simulink model "ASDdc_SelectParameter"  (R2016b)
settings: configuration reference "CodeGenConfigSet" (kept outside this file)
values from neighbouring files (symbols this model uses):
  ASDdc_DT1GovGear0_CUR = Calibration.Parameter    [init_ASDdc_SelectParameter.m]    (also in init_ASDdc_SelectParameter_SIL.m = Simulink.Parameter)
  ASDdc_DT1GovGear0_CURX = Calibration.Parameter    [init_ASDdc_SelectParameter.m]    (also in init_ASDdc_SelectParameter_SIL.m = Simulink.Parameter)
  ASDdc_DT1GovGear1_CUR = Calibration.Parameter    [init_ASDdc_SelectParameter.m]    (also in init_ASDdc_SelectParameter_SIL.m = Simulink.Parameter)
  ASDdc_DT1GovGear1_CURX = Calibration.Parameter    [init_ASDdc_SelectParameter.m]    (also in init_ASDdc_SelectParameter_SIL.m = Simulink.Parameter)
  ASDdc_DT1GovGear2_CUR = Calibration.Parameter    [init_ASDdc_SelectParameter.m]    (also in init_ASDdc_SelectParameter_SIL.m = Simulink.Parameter)
  ASDdc_DT1GovGear2_CURX = Calibration.Parameter    [init_ASDdc_SelectParameter.m]    (also in init_ASDdc_SelectParameter_SIL.m = Simulink.Parameter)
  ASDdc_DT1GovGear3_CUR = Calibration.Parameter    [init_ASDdc_SelectParameter.m]    (also in init_ASDdc_SelectParameter_SIL.m = Simulink.Parameter)
  ASDdc_DT1GovGear3_CURX = Calibration.Parameter    [init_ASDdc_SelectParameter.m]    (also in init_ASDdc_SelectParameter_SIL.m = Simulink.Parameter)
  ASDdc_DT1GovGear4_CUR = Calibration.Parameter    [init_ASDdc_SelectParameter.m]    (also in init_ASDdc_SelectParameter_SIL.m = Simulink.Parameter)
  ASDdc_DT1GovGear4_CURX = Calibration.Parameter    [init_ASDdc_SelectParameter.m]    (also in init_ASDdc_SelectParameter_SIL.m = Simulink.Parameter)
  ASDdc_DT1GovGear5_CUR = Calibration.Parameter    [init_ASDdc_SelectParameter.m]    (also in init_ASDdc_SelectParameter_SIL.m = Simulink.Parameter)
  ASDdc_DT1GovGear5_CURX = Calibration.Parameter    [init_ASDdc_SelectParameter.m]    (also in init_ASDdc_SelectParameter_SIL.m = Simulink.Parameter)
  ASDdc_KdGovGear0_CUR = Calibration.Parameter    [init_ASDdc_SelectParameter.m]    (also in init_ASDdc_SelectParameter_SIL.m = Simulink.Parameter)
  ASDdc_KdGovGear0_CURX = Calibration.Parameter    [init_ASDdc_SelectParameter.m]    (also in init_ASDdc_SelectParameter_SIL.m = Simulink.Parameter)
  ASDdc_KdGovGear1_CUR = Calibration.Parameter    [init_ASDdc_SelectParameter.m]    (also in init_ASDdc_SelectParameter_SIL.m = Simulink.Parameter)
  ASDdc_KdGovGear1_CURX = Calibration.Parameter    [init_ASDdc_SelectParameter.m]    (also in init_ASDdc_SelectParameter_SIL.m = Simulink.Parameter)
  ASDdc_KdGovGear2_CUR = Calibration.Parameter    [init_ASDdc_SelectParameter.m]    (also in init_ASDdc_SelectParameter_SIL.m = Simulink.Parameter)
  ASDdc_KdGovGear2_CURX = Calibration.Parameter    [init_ASDdc_SelectParameter.m]    (also in init_ASDdc_SelectParameter_SIL.m = Simulink.Parameter)
  ASDdc_KdGovGear3_CUR = Calibration.Parameter    [init_ASDdc_SelectParameter.m]    (also in init_ASDdc_SelectParameter_SIL.m = Simulink.Parameter)
  ASDdc_KdGovGear3_CURX = Calibration.Parameter    [init_ASDdc_SelectParameter.m]    (also in init_ASDdc_SelectParameter_SIL.m = Simulink.Parameter)
  ASDdc_KdGovGear4_CUR = Calibration.Parameter    [init_ASDdc_SelectParameter.m]    (also in init_ASDdc_SelectParameter_SIL.m = Simulink.Parameter)
  ASDdc_KdGovGear4_CURX = Calibration.Parameter    [init_ASDdc_SelectParameter.m]    (also in init_ASDdc_SelectParameter_SIL.m = Simulink.Parameter)
  ASDdc_KdGovGear5_CUR = Calibration.Parameter    [init_ASDdc_SelectParameter.m]    (also in init_ASDdc_SelectParameter_SIL.m = Simulink.Parameter)
  ASDdc_KdGovGear5_CURX = Calibration.Parameter    [init_ASDdc_SelectParameter.m]    (also in init_ASDdc_SelectParameter_SIL.m = Simulink.Parameter)
settings Model: Creator=lenovo  LastModifiedBy=wangrui
settings ConfigSetRef: SourceLocation=Base Workspace

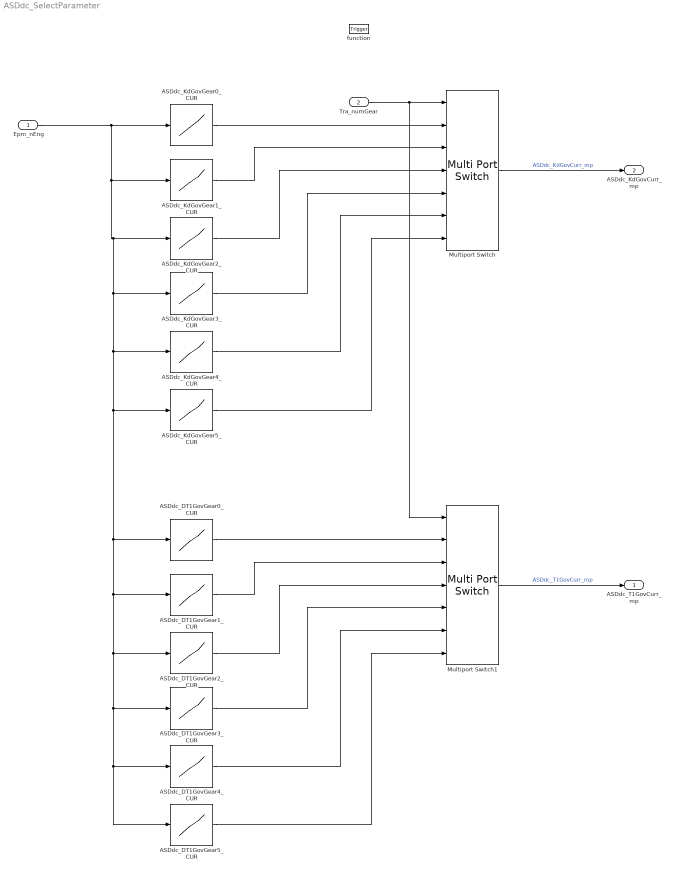
== system ASDdc_SelectParameter ==
  Epm_nEng : Inport  Tag=rpm  Description=Engine speed  OutMin=0  OutMax=6000  OutDataTypeStr=EngSpeed_rpm
  Tra_numGear : Inport  Description=Current gear information  Port=2  OutMin=-128  OutMax=127  OutDataTypeStr=Tra_num
  function : TriggerPort  TriggerType=function-call  VariantControl=Variant
  ASDdc_DT1GovGear0_CUR : Lookup_n-D  NumberOfTableDimensions=1  BreakpointsForDimension1=ASDdc_DT1GovGear0_CURX  IndexSearchMethod=Linear search  BeginIndexSearchUsingPreviousIndexResult=on  Table=ASDdc_DT1GovGear0_CUR  ExtrapMethod=Clip  UseLastTableValue=on  InternalRulePriority=Speed  OutDataTypeStr=Inherit: Inherit via back propagation  SaturateOnIntegerOverflow=on
  ASDdc_DT1GovGear1_CUR : Lookup_n-D  NumberOfTableDimensions=1  BreakpointsForDimension1=ASDdc_DT1GovGear1_CURX  IndexSearchMethod=Linear search  BeginIndexSearchUsingPreviousIndexResult=on  Table=ASDdc_DT1GovGear1_CUR  ExtrapMethod=Clip  UseLastTableValue=on  InternalRulePriority=Speed  OutDataTypeStr=Inherit: Inherit via back propagation  SaturateOnIntegerOverflow=on
  ASDdc_DT1GovGear2_CUR : Lookup_n-D  NumberOfTableDimensions=1  BreakpointsForDimension1=ASDdc_DT1GovGear2_CURX  IndexSearchMethod=Linear search  BeginIndexSearchUsingPreviousIndexResult=on  Table=ASDdc_DT1GovGear2_CUR  ExtrapMethod=Clip  UseLastTableValue=on  InternalRulePriority=Speed  OutDataTypeStr=Inherit: Inherit via back propagation  SaturateOnIntegerOverflow=on
  ASDdc_DT1GovGear3_CUR : Lookup_n-D  NumberOfTableDimensions=1  BreakpointsForDimension1=ASDdc_DT1GovGear3_CURX  IndexSearchMethod=Linear search  BeginIndexSearchUsingPreviousIndexResult=on  Table=ASDdc_DT1GovGear3_CUR  ExtrapMethod=Clip  UseLastTableValue=on  InternalRulePriority=Speed  OutDataTypeStr=Inherit: Inherit via back propagation  SaturateOnIntegerOverflow=on
  ASDdc_DT1GovGear4_CUR : Lookup_n-D  NumberOfTableDimensions=1  BreakpointsForDimension1=ASDdc_DT1GovGear4_CURX  IndexSearchMethod=Linear search  BeginIndexSearchUsingPreviousIndexResult=on  Table=ASDdc_DT1GovGear4_CUR  ExtrapMethod=Clip  UseLastTableValue=on  InternalRulePriority=Speed  OutDataTypeStr=Inherit: Inherit via back propagation  SaturateOnIntegerOverflow=on
  ASDdc_DT1GovGear5_CUR : Lookup_n-D  NumberOfTableDimensions=1  BreakpointsForDimension1=ASDdc_DT1GovGear5_CURX  IndexSearchMethod=Linear search  BeginIndexSearchUsingPreviousIndexResult=on  Table=ASDdc_DT1GovGear5_CUR  ExtrapMethod=Clip  UseLastTableValue=on  InternalRulePriority=Speed  OutDataTypeStr=Inherit: Inherit via back propagation  SaturateOnIntegerOverflow=on
  ASDdc_KdGovGear0_CUR : Lookup_n-D  NumberOfTableDimensions=1  BreakpointsForDimension1=ASDdc_KdGovGear0_CURX  IndexSearchMethod=Linear search  BeginIndexSearchUsingPreviousIndexResult=on  Table=ASDdc_KdGovGear0_CUR  ExtrapMethod=Clip  UseLastTableValue=on  InternalRulePriority=Speed  OutDataTypeStr=Inherit: Inherit via back propagation  SaturateOnIntegerOverflow=on
  ASDdc_KdGovGear1_CUR : Lookup_n-D  NumberOfTableDimensions=1  BreakpointsForDimension1=ASDdc_KdGovGear1_CURX  IndexSearchMethod=Linear search  BeginIndexSearchUsingPreviousIndexResult=on  Table=ASDdc_KdGovGear1_CUR  ExtrapMethod=Clip  UseLastTableValue=on  InternalRulePriority=Speed  OutDataTypeStr=Inherit: Inherit via back propagation  SaturateOnIntegerOverflow=on
  ASDdc_KdGovGear2_CUR : Lookup_n-D  NumberOfTableDimensions=1  BreakpointsForDimension1=ASDdc_KdGovGear2_CURX  IndexSearchMethod=Linear search  BeginIndexSearchUsingPreviousIndexResult=on  Table=ASDdc_KdGovGear2_CUR  ExtrapMethod=Clip  UseLastTableValue=on  InternalRulePriority=Speed  OutDataTypeStr=Inherit: Inherit via back propagation  SaturateOnIntegerOverflow=on
  ASDdc_KdGovGear3_CUR : Lookup_n-D  NumberOfTableDimensions=1  BreakpointsForDimension1=ASDdc_KdGovGear3_CURX  IndexSearchMethod=Linear search  BeginIndexSearchUsingPreviousIndexResult=on  Table=ASDdc_KdGovGear3_CUR  ExtrapMethod=Clip  UseLastTableValue=on  InternalRulePriority=Speed  OutDataTypeStr=Inherit: Inherit via back propagation  SaturateOnIntegerOverflow=on
  ASDdc_KdGovGear4_CUR : Lookup_n-D  NumberOfTableDimensions=1  BreakpointsForDimension1=ASDdc_KdGovGear4_CURX  IndexSearchMethod=Linear search  BeginIndexSearchUsingPreviousIndexResult=on  Table=ASDdc_KdGovGear4_CUR  ExtrapMethod=Clip  UseLastTableValue=on  InternalRulePriority=Speed  OutDataTypeStr=Inherit: Inherit via back propagation  SaturateOnIntegerOverflow=on
  ASDdc_KdGovGear5_CUR : Lookup_n-D  NumberOfTableDimensions=1  BreakpointsForDimension1=ASDdc_KdGovGear5_CURX  IndexSearchMethod=Linear search  BeginIndexSearchUsingPreviousIndexResult=on  Table=ASDdc_KdGovGear5_CUR  ExtrapMethod=Clip  UseLastTableValue=on  InternalRulePriority=Speed  OutDataTypeStr=Inherit: Inherit via back propagation  SaturateOnIntegerOverflow=on
  Multiport Switch : MultiPortSwitch  DataPortOrder=Zero-based contiguous  Inputs=6
  Multiport Switch1 : MultiPortSwitch  DataPortOrder=Zero-based contiguous  Inputs=6
  ASDdc_T1GovCurr_mp : Outport  Tag=ms  Description=Current parameter T1 for ASD disturbance compensator  OutMin=0  OutMax=65535  OutDataTypeStr=RailDT1_ms
  ASDdc_KdGovCurr_mp : Outport  Description=Current parameter Kd for ASD disturbance compensator  Port=2  OutMin=0  OutMax=15  OutDataTypeStr=Pid_Kp_Kd
  wires:
  Multiport Switch1/1 -> ASDdc_T1GovCurr_mp/1  "ASDdc_T1GovCurr_mp"
  Multiport Switch/1 -> ASDdc_KdGovCurr_mp/1  "ASDdc_KdGovCurr_mp"
  Tra_numGear/1 -> Multiport Switch1/1, Multiport Switch/1
  ASDdc_KdGovGear0_CUR/1 -> Multiport Switch/2
  ASDdc_KdGovGear1_CUR/1 -> Multiport Switch/3
  ASDdc_KdGovGear2_CUR/1 -> Multiport Switch/4
  ASDdc_KdGovGear3_CUR/1 -> Multiport Switch/5
  ASDdc_KdGovGear4_CUR/1 -> Multiport Switch/6
  ASDdc_KdGovGear5_CUR/1 -> Multiport Switch/7
  ASDdc_DT1GovGear0_CUR/1 -> Multiport Switch1/2
  Epm_nEng/1 -> ASDdc_DT1GovGear4_CUR/1, ASDdc_DT1GovGear5_CUR/1, ASDdc_DT1GovGear3_CUR/1, ASDdc_DT1GovGear2_CUR/1, ASDdc_DT1GovGear1_CUR/1, ASDdc_DT1GovGear0_CUR/1, ASDdc_KdGovGear5_CUR/1, ASDdc_KdGovGear4_CUR/1, ASDdc_KdGovGear3_CUR/1, ASDdc_KdGovGear2_CUR/1, ASDdc_KdGovGear1_CUR/1, ASDdc_KdGovGear0_CUR/1
  ASDdc_DT1GovGear1_CUR/1 -> Multiport Switch1/3
  ASDdc_DT1GovGear2_CUR/1 -> Multiport Switch1/4
  ASDdc_DT1GovGear3_CUR/1 -> Multiport Switch1/5
  ASDdc_DT1GovGear4_CUR/1 -> Multiport Switch1/6
  ASDdc_DT1GovGear5_CUR/1 -> Multiport Switch1/7
